simulink model "ieee30"  (R2017a)
settings: Solver=VariableStepDiscrete  StartTime=0.0  StopTime=0.012  MaxStep=1e-4  RelTol=1e-3
undefined symbols (not defined in the file): Angle, Magnitude
libraries: powerlib x548
(part 2 of 4)

== system ieee30/Bus1 ==
  G1 : powerlib/Measurements/Three-Phase V-I Measurement  VoltageMeasurement=no  SetLabelV=off  LabelV=V1  Vpu=off  VpuLL=off  CurrentMeasurement=no  SetLabelI=off  LabelI=I12  Ipu=off  Pbase=100e6  Vbase=500e3  OutputType=Complex  PhasorSimulation=on  PSBequivalent=0
  I13 : powerlib/Measurements/Three-Phase V-I Measurement  VoltageMeasurement=no  SetLabelV=off  LabelV=V1  Vpu=off  VpuLL=off  CurrentMeasurement=yes  SetLabelI=on  LabelI=I13  Ipu=off  Pbase=100e6  Vbase=500e3  OutputType=Magnitude-Angle  PhasorSimulation=on  PSBequivalent=0
  To Workspace2 : ToWorkspace  VariableName=I13  SaveFormat=Timeseries  SampleTime=0.01
  To Workspace3 : ToWorkspace  VariableName=I12  SaveFormat=Timeseries  SampleTime=0.01
  To Workspace4 : ToWorkspace  VariableName=V1  SaveFormat=Timeseries  SampleTime=0.01
  V1 I12 : powerlib/Measurements/Three-Phase V-I Measurement  VoltageMeasurement=phase-to-phase  SetLabelV=on  LabelV=V1  Vpu=off  VpuLL=off  CurrentMeasurement=yes  SetLabelI=on  LabelI=I12  Ipu=off  Pbase=100e6  Vbase=500e3  OutputType=Magnitude-Angle  PhasorSimulation=on  PSBequivalent=0
  G1A : PMIOPort  Port=1  Side=Left
  G1B : PMIOPort  Port=2  Side=Left
  G1C : PMIOPort  Port=3  Side=Left
  I13A : PMIOPort  Port=4  Side=Right
  I13B : PMIOPort  Port=5  Side=Right
  I13C : PMIOPort  Port=6  Side=Right
  I12C : PMIOPort  Port=7  Side=Right
  I12B : PMIOPort  Port=8  Side=Right
  I12A : PMIOPort  Port=9  Side=Right
  wires:
  [V1] -> To Workspace4/1
  [I12] -> To Workspace3/1
  [I13] -> To Workspace2/1
  connections:
  I13/LConn1 -- V1 I12/LConn1 -- G1/LConn1
  I13/LConn2 -- G1/LConn2 -- V1 I12/LConn2
  I13/LConn3 -- V1 I12/LConn3 -- G1/LConn3
  V1 I12/RConn1 -- I12A/RConn1
  V1 I12/RConn2 -- I12B/RConn1
  I12C/RConn1 -- V1 I12/RConn3
  I13/RConn3 -- I13C/RConn1
  I13/RConn1 -- I13A/RConn1
  I13/RConn2 -- I13B/RConn1
  G1B/RConn1 -- G1/RConn2
  G1A/RConn1 -- G1/RConn1
  G1C/RConn1 -- G1/RConn3

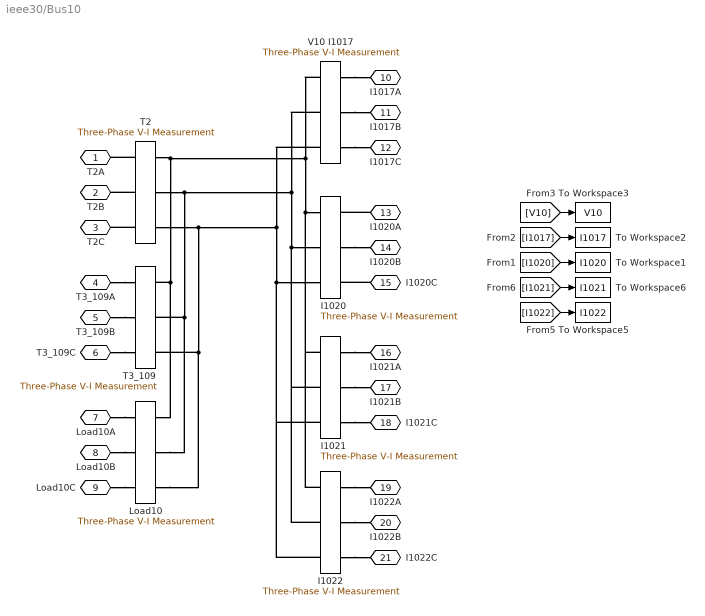
== system ieee30/Bus10 ==
  I1020 : powerlib/Measurements/Three-Phase V-I Measurement  VoltageMeasurement=no  SetLabelV=off  LabelV=V10  Vpu=off  VpuLL=off  CurrentMeasurement=yes  SetLabelI=on  LabelI=I1020  Ipu=off  Pbase=100e6  Vbase=500e3  OutputType=Magnitude-Angle  PhasorSimulation=on  PSBequivalent=0
  I1021 : powerlib/Measurements/Three-Phase V-I Measurement  VoltageMeasurement=no  SetLabelV=off  LabelV=V10  Vpu=off  VpuLL=off  CurrentMeasurement=yes  SetLabelI=on  LabelI=I1021  Ipu=off  Pbase=100e6  Vbase=500e3  OutputType=Magnitude-Angle  PhasorSimulation=on  PSBequivalent=0
  I1022 : powerlib/Measurements/Three-Phase V-I Measurement  VoltageMeasurement=no  SetLabelV=off  LabelV=V10  Vpu=off  VpuLL=off  CurrentMeasurement=yes  SetLabelI=on  LabelI=I1022  Ipu=off  Pbase=100e6  Vbase=500e3  OutputType=Magnitude-Angle  PhasorSimulation=on  PSBequivalent=0
  Load10 : powerlib/Measurements/Three-Phase V-I Measurement  VoltageMeasurement=no  SetLabelV=off  LabelV=Vabc  Vpu=off  VpuLL=off  CurrentMeasurement=no  SetLabelI=off  LabelI=Iabc  Ipu=off  Pbase=100e6  Vbase=500e3  OutputType=Complex  PhasorSimulation=on  PSBequivalent=0
  T2 : powerlib/Measurements/Three-Phase V-I Measurement  VoltageMeasurement=no  SetLabelV=off  LabelV=Vabc  Vpu=off  VpuLL=off  CurrentMeasurement=no  SetLabelI=off  LabelI=Iabc  Ipu=off  Pbase=100e6  Vbase=500e3  OutputType=Complex  PhasorSimulation=on  PSBequivalent=0
  T3_109 : powerlib/Measurements/Three-Phase V-I Measurement  VoltageMeasurement=no  SetLabelV=off  LabelV=Vabc  Vpu=off  VpuLL=off  CurrentMeasurement=no  SetLabelI=off  LabelI=Iabc  Ipu=off  Pbase=100e6  Vbase=500e3  OutputType=Complex  PhasorSimulation=on  PSBequivalent=0
  To Workspace1 : ToWorkspace  VariableName=I1020  SaveFormat=Timeseries  SampleTime=0.01
  To Workspace2 : ToWorkspace  VariableName=I1017  SaveFormat=Timeseries  SampleTime=0.01
  To Workspace3 : ToWorkspace  VariableName=V10  SaveFormat=Timeseries  SampleTime=0.01
  To Workspace5 : ToWorkspace  VariableName=I1022  SaveFormat=Timeseries  SampleTime=0.01
  To Workspace6 : ToWorkspace  VariableName=I1021  SaveFormat=Timeseries  SampleTime=0.01
  V10 I1017 : powerlib/Measurements/Three-Phase V-I Measurement  VoltageMeasurement=phase-to-phase  SetLabelV=on  LabelV=V10  Vpu=off  VpuLL=off  CurrentMeasurement=yes  SetLabelI=on  LabelI=I1017  Ipu=off  Pbase=100e6  Vbase=500e3  OutputType=Magnitude-Angle  PhasorSimulation=on  PSBequivalent=0
  T2A : PMIOPort  Port=1  Side=Left
  T2B : PMIOPort  Port=2  Side=Left
  T2C : PMIOPort  Port=3  Side=Left
  T3_109A : PMIOPort  Port=4  Side=Left
  T3_109B : PMIOPort  Port=5  Side=Left
  T3_109C : PMIOPort  Port=6  Side=Left
  Load10A : PMIOPort  Port=7  Side=Left
  Load10B : PMIOPort  Port=8  Side=Left
  Load10C : PMIOPort  Port=9  Side=Left
  I1017A : PMIOPort  Port=10  Side=Right
  I1017B : PMIOPort  Port=11  Side=Right
  I1017C : PMIOPort  Port=12  Side=Right
  I1020A : PMIOPort  Port=13  Side=Right
  I1020B : PMIOPort  Port=14  Side=Right
  I1020C : PMIOPort  Port=15  Side=Right
  I1021A : PMIOPort  Port=16  Side=Right
  I1021B : PMIOPort  Port=17  Side=Right
  I1021C : PMIOPort  Port=18  Side=Right
  I1022A : PMIOPort  Port=19  Side=Right
  I1022B : PMIOPort  Port=20  Side=Right
  I1022C : PMIOPort  Port=21  Side=Right
  wires:
  [I1020] -> To Workspace1/1
  [I1017] -> To Workspace2/1
  [I1022] -> To Workspace5/1
  [I1021] -> To Workspace6/1
  [V10] -> To Workspace3/1
  connections:
  T2/RConn3 -- T2C/RConn1
  T2/RConn1 -- T2A/RConn1
  T2/RConn2 -- T2B/RConn1
  T2/LConn1 -- I1022/LConn1 -- I1021/LConn1 -- I1020/LConn1 -- V10 I1017/LConn1 -- Load10/LConn1 -- T3_109/LConn1
  T2/LConn2 -- I1021/LConn2 -- I1022/LConn2 -- I1020/LConn2 -- V10 I1017/LConn2 -- Load10/LConn2 -- T3_109/LConn2
  T2/LConn3 -- Load10/LConn3 -- T3_109/LConn3 -- I1021/LConn3 -- I1022/LConn3 -- I1020/LConn3 -- V10 I1017/LConn3
  T3_109A/RConn1 -- T3_109/RConn1
  T3_109B/RConn1 -- T3_109/RConn2
  T3_109C/RConn1 -- T3_109/RConn3
  Load10C/RConn1 -- Load10/RConn3
  Load10B/RConn1 -- Load10/RConn2
  Load10A/RConn1 -- Load10/RConn1
  V10 I1017/RConn1 -- I1017A/RConn1
  V10 I1017/RConn3 -- I1017C/RConn1
  V10 I1017/RConn2 -- I1017B/RConn1
  I1020A/RConn1 -- I1020/RConn1
  I1020/RConn2 -- I1020B/RConn1
  I1020C/RConn1 -- I1020/RConn3
  I1021/RConn1 -- I1021A/RConn1
  I1021/RConn2 -- I1021B/RConn1
  I1021/RConn3 -- I1021C/RConn1
  I1022/RConn2 -- I1022B/RConn1
  I1022/RConn1 -- I1022A/RConn1
  I1022/RConn3 -- I1022C/RConn1

== system ieee30/Bus11 ==
  G11 : powerlib/Measurements/Three-Phase V-I Measurement  VoltageMeasurement=no  SetLabelV=off  LabelV=Vabc  Vpu=off  VpuLL=off  CurrentMeasurement=no  SetLabelI=off  LabelI=Iabc  Ipu=off  Pbase=100e6  Vbase=500e3  OutputType=Complex  PhasorSimulation=on  PSBequivalent=0
  T3_911 : powerlib/Measurements/Three-Phase V-I Measurement  VoltageMeasurement=no  SetLabelV=off  LabelV=Vabc  Vpu=off  VpuLL=off  CurrentMeasurement=no  SetLabelI=off  LabelI=Iabc  Ipu=off  Pbase=100e6  Vbase=500e3  OutputType=Complex  PhasorSimulation=on  PSBequivalent=0
  T3_911A : PMIOPort  Port=1  Side=Left
  T3_911B : PMIOPort  Port=2  Side=Left
  T3_911C : PMIOPort  Port=3  Side=Left
  G11A : PMIOPort  Port=4  Side=Right
  G11B : PMIOPort  Port=5  Side=Right
  G11C : PMIOPort  Port=6  Side=Right
  connections:
  T3_911/RConn1 -- T3_911A/RConn1
  T3_911/RConn2 -- T3_911B/RConn1
  G11/RConn3 -- G11C/RConn1
  G11/RConn2 -- G11B/RConn1
  G11/RConn1 -- G11A/RConn1
  T3_911/RConn3 -- T3_911C/RConn1
  T3_911/LConn1 -- G11/LConn1
  T3_911/LConn2 -- G11/LConn2
  T3_911/LConn3 -- G11/LConn3

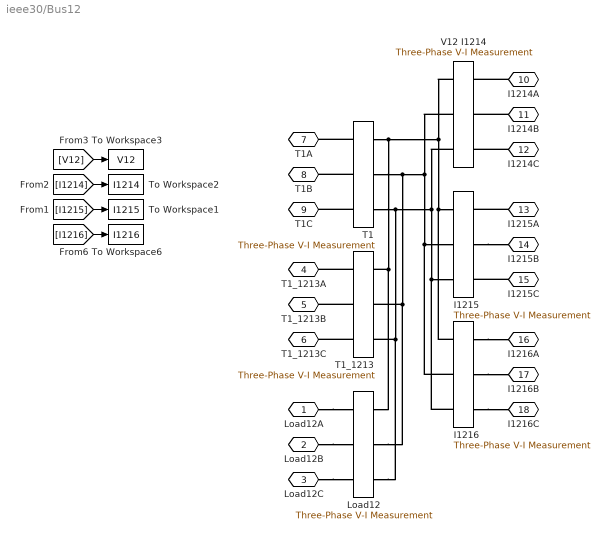
== system ieee30/Bus12 ==
  I1215 : powerlib/Measurements/Three-Phase V-I Measurement  VoltageMeasurement=no  SetLabelV=off  LabelV=V12  Vpu=off  VpuLL=off  CurrentMeasurement=yes  SetLabelI=on  LabelI=I1215  Ipu=off  Pbase=100e6  Vbase=500e3  OutputType=Magnitude-Angle  PhasorSimulation=on  PSBequivalent=0
  I1216 : powerlib/Measurements/Three-Phase V-I Measurement  VoltageMeasurement=no  SetLabelV=off  LabelV=V12  Vpu=off  VpuLL=off  CurrentMeasurement=yes  SetLabelI=on  LabelI=I1216  Ipu=off  Pbase=100e6  Vbase=500e3  OutputType=Magnitude-Angle  PhasorSimulation=on  PSBequivalent=0
  Load12 : powerlib/Measurements/Three-Phase V-I Measurement  VoltageMeasurement=no  SetLabelV=off  LabelV=V12  Vpu=off  VpuLL=off  CurrentMeasurement=no  SetLabelI=off  LabelI=I1214  Ipu=off  Pbase=100e6  Vbase=500e3  OutputType=Complex  PhasorSimulation=on  PSBequivalent=0
  T1 : powerlib/Measurements/Three-Phase V-I Measurement  VoltageMeasurement=no  SetLabelV=off  LabelV=V12  Vpu=off  VpuLL=off  CurrentMeasurement=no  SetLabelI=off  LabelI=I1214  Ipu=off  Pbase=100e6  Vbase=500e3  OutputType=Complex  PhasorSimulation=on  PSBequivalent=0
  T1_1213 : powerlib/Measurements/Three-Phase V-I Measurement  VoltageMeasurement=no  SetLabelV=off  LabelV=V12  Vpu=off  VpuLL=off  CurrentMeasurement=no  SetLabelI=off  LabelI=I1214  Ipu=off  Pbase=100e6  Vbase=500e3  OutputType=Complex  PhasorSimulation=on  PSBequivalent=0
  To Workspace1 : ToWorkspace  VariableName=I1215  SaveFormat=Timeseries  SampleTime=0.01
  To Workspace2 : ToWorkspace  VariableName=I1214  SaveFormat=Timeseries  SampleTime=0.01
  To Workspace3 : ToWorkspace  VariableName=V12  SaveFormat=Timeseries  SampleTime=0.01
  To Workspace6 : ToWorkspace  VariableName=I1216  SaveFormat=Timeseries  SampleTime=0.01
  V12 I1214 : powerlib/Measurements/Three-Phase V-I Measurement  VoltageMeasurement=phase-to-phase  SetLabelV=on  LabelV=V12  Vpu=off  VpuLL=off  CurrentMeasurement=yes  SetLabelI=on  LabelI=I1214  Ipu=off  Pbase=100e6  Vbase=500e3  OutputType=Magnitude-Angle  PhasorSimulation=on  PSBequivalent=0
  Load12A : PMIOPort  Port=1  Side=Left
  Load12B : PMIOPort  Port=2  Side=Left
  Load12C : PMIOPort  Port=3  Side=Left
  T1_1213A : PMIOPort  Port=4  Side=Left
  T1_1213B : PMIOPort  Port=5  Side=Left
  T1_1213C : PMIOPort  Port=6  Side=Left
  T1A : PMIOPort  Port=7  Side=Left
  T1B : PMIOPort  Port=8  Side=Left
  T1C : PMIOPort  Port=9  Side=Left
  I1214A : PMIOPort  Port=10  Side=Right
  I1214B : PMIOPort  Port=11  Side=Right
  I1214C : PMIOPort  Port=12  Side=Right
  I1215A : PMIOPort  Port=13  Side=Right
  I1215B : PMIOPort  Port=14  Side=Right
  I1215C : PMIOPort  Port=15  Side=Right
  I1216A : PMIOPort  Port=16  Side=Right
  I1216B : PMIOPort  Port=17  Side=Right
  I1216C : PMIOPort  Port=18  Side=Right
  wires:
  [I1215] -> To Workspace1/1
  [I1214] -> To Workspace2/1
  [I1216] -> To Workspace6/1
  [V12] -> To Workspace3/1
  connections:
  I1214C/RConn1 -- V12 I1214/RConn3
  I1214A/RConn1 -- V12 I1214/RConn1
  I1214B/RConn1 -- V12 I1214/RConn2
  T1/RConn2 -- T1B/RConn1
  T1/RConn3 -- T1C/RConn1
  T1/RConn1 -- T1A/RConn1
  T1/LConn1 -- Load12/LConn1 -- T1_1213/LConn1 -- I1216/LConn1 -- I1215/LConn1 -- V12 I1214/LConn1
  T1/LConn2 -- T1_1213/LConn2 -- Load12/LConn2 -- I1216/LConn2 -- I1215/LConn2 -- V12 I1214/LConn2
  T1/LConn3 -- I1216/LConn3 -- I1215/LConn3 -- V12 I1214/LConn3 -- T1_1213/LConn3 -- Load12/LConn3
  T1_1213/RConn3 -- T1_1213C/RConn1
  T1_1213/RConn2 -- T1_1213B/RConn1
  T1_1213/RConn1 -- T1_1213A/RConn1
  I1215A/RConn1 -- I1215/RConn1
  I1215/RConn2 -- I1215B/RConn1
  I1215C/RConn1 -- I1215/RConn3
  I1216/RConn1 -- I1216A/RConn1
  I1216/RConn3 -- I1216C/RConn1
  I1216/RConn2 -- I1216B/RConn1
  Load12A/RConn1 -- Load12/RConn1
  Load12B/RConn1 -- Load12/RConn2
  Load12C/RConn1 -- Load12/RConn3

== system ieee30/Bus13 ==
  G13 : powerlib/Measurements/Three-Phase V-I Measurement  VoltageMeasurement=no  SetLabelV=off  LabelV=Vabc  Vpu=off  VpuLL=off  CurrentMeasurement=no  SetLabelI=off  LabelI=Iabc  Ipu=off  Pbase=100e6  Vbase=500e3  OutputType=Complex  PhasorSimulation=on  PSBequivalent=0
  T1_1213 : powerlib/Measurements/Three-Phase V-I Measurement  VoltageMeasurement=no  SetLabelV=off  LabelV=Vabc  Vpu=off  VpuLL=off  CurrentMeasurement=no  SetLabelI=off  LabelI=Iabc  Ipu=off  Pbase=100e6  Vbase=500e3  OutputType=Complex  PhasorSimulation=on  PSBequivalent=0
  T1_1213A : PMIOPort  Port=1  Side=Left
  T1_1213B : PMIOPort  Port=2  Side=Left
  T1_1213C : PMIOPort  Port=3  Side=Left
  G13A : PMIOPort  Port=4  Side=Right
  G13B : PMIOPort  Port=5  Side=Right
  G13C : PMIOPort  Port=6  Side=Right
  connections:
  G13/RConn3 -- G13C/RConn1
  T1_1213/RConn3 -- T1_1213C/RConn1
  T1_1213/RConn1 -- T1_1213A/RConn1
  G13/RConn2 -- G13B/RConn1
  G13/RConn1 -- G13A/RConn1
  T1_1213/RConn2 -- T1_1213B/RConn1
  G13/LConn1 -- T1_1213/LConn1
  G13/LConn2 -- T1_1213/LConn2
  G13/LConn3 -- T1_1213/LConn3

== system ieee30/Bus14 ==
  I1415 : powerlib/Measurements/Three-Phase V-I Measurement  VoltageMeasurement=no  SetLabelV=off  LabelV=Vabc  Vpu=off  VpuLL=off  CurrentMeasurement=yes  SetLabelI=on  LabelI=I1415  Ipu=off  Pbase=100e6  Vbase=500e3  OutputType=Magnitude-Angle  PhasorSimulation=on  PSBequivalent=0
  Load14 : powerlib/Measurements/Three-Phase V-I Measurement  VoltageMeasurement=no  SetLabelV=off  LabelV=Vabc  Vpu=off  VpuLL=off  CurrentMeasurement=no  SetLabelI=off  LabelI=I1415  Ipu=off  Pbase=100e6  Vbase=500e3  OutputType=Complex  PhasorSimulation=on  PSBequivalent=0
  To Workspace1 : ToWorkspace  VariableName=I1415  SaveFormat=Timeseries  SampleTime=0.01
  To Workspace2 : ToWorkspace  VariableName=I1412  SaveFormat=Timeseries  SampleTime=0.01
  To Workspace3 : ToWorkspace  VariableName=V14  SaveFormat=Timeseries  SampleTime=0.01
  V14 I1412 : powerlib/Measurements/Three-Phase V-I Measurement  VoltageMeasurement=phase-to-phase  SetLabelV=on  LabelV=V14  Vpu=off  VpuLL=off  CurrentMeasurement=yes  SetLabelI=on  LabelI=I1412  Ipu=off  Pbase=100e6  Vbase=500e3  OutputType=Magnitude-Angle  PhasorSimulation=on  PSBequivalent=0
  Load14A : PMIOPort  Port=1  Side=Left
  Load14B : PMIOPort  Port=2  Side=Left
  Load14C : PMIOPort  Port=3  Side=Left
  I1412A : PMIOPort  Port=4  Side=Left
  I1412B : PMIOPort  Port=5  Side=Left
  I1412C : PMIOPort  Port=6  Side=Left
  I1415A : PMIOPort  Port=7  Side=Right
  I1415B : PMIOPort  Port=8  Side=Right
  I1415C : PMIOPort  Port=9  Side=Right
  wires:
  [V14] -> To Workspace3/1
  [I1415] -> To Workspace1/1
  [I1412] -> To Workspace2/1
  connections:
  I1415/RConn3 -- I1415C/RConn1
  V14 I1412/RConn3 -- I1412C/RConn1
  V14 I1412/RConn2 -- I1412B/RConn1
  I1415/RConn2 -- I1415B/RConn1
  V14 I1412/RConn1 -- I1412A/RConn1
  I1415/RConn1 -- I1415A/RConn1
  V14 I1412/LConn1 -- Load14/LConn1 -- I1415/LConn1
  V14 I1412/LConn2 -- I1415/LConn2 -- Load14/LConn2
  V14 I1412/LConn3 -- I1415/LConn3 -- Load14/LConn3
  Load14A/RConn1 -- Load14/RConn1
  Load14/RConn2 -- Load14B/RConn1
  Load14C/RConn1 -- Load14/RConn3

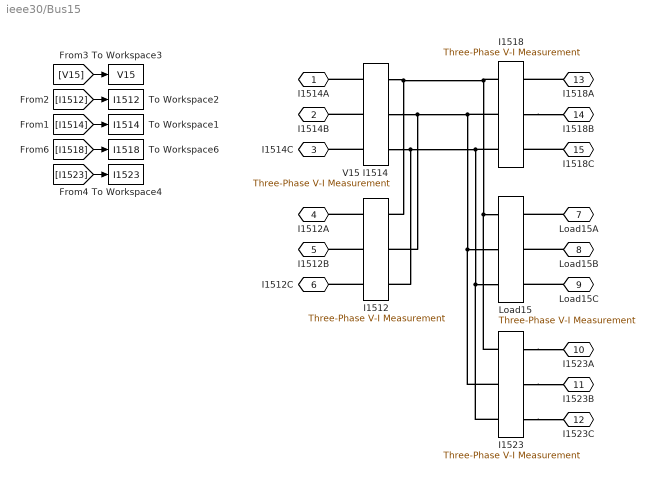
== system ieee30/Bus15 ==
  I1512 : powerlib/Measurements/Three-Phase V-I Measurement  VoltageMeasurement=no  SetLabelV=off  LabelV=V15  Vpu=off  VpuLL=off  CurrentMeasurement=yes  SetLabelI=on  LabelI=I1512  Ipu=off  Pbase=100e6  Vbase=500e3  OutputType=Magnitude-Angle  PhasorSimulation=on  PSBequivalent=0
  I1518 : powerlib/Measurements/Three-Phase V-I Measurement  VoltageMeasurement=no  SetLabelV=off  LabelV=Vabc  Vpu=off  VpuLL=off  CurrentMeasurement=yes  SetLabelI=on  LabelI=I1518  Ipu=off  Pbase=100e6  Vbase=500e3  OutputType=Magnitude-Angle  PhasorSimulation=on  PSBequivalent=0
  I1523 : powerlib/Measurements/Three-Phase V-I Measurement  VoltageMeasurement=no  SetLabelV=off  LabelV=Vabc  Vpu=off  VpuLL=off  CurrentMeasurement=yes  SetLabelI=on  LabelI=I1523  Ipu=off  Pbase=100e6  Vbase=500e3  OutputType=Magnitude-Angle  PhasorSimulation=on  PSBequivalent=0
  Load15 : powerlib/Measurements/Three-Phase V-I Measurement  VoltageMeasurement=no  SetLabelV=off  LabelV=Vabc  Vpu=off  VpuLL=off  CurrentMeasurement=no  SetLabelI=off  LabelI=Iabc  Ipu=off  Pbase=100e6  Vbase=500e3  OutputType=Complex  PhasorSimulation=on  PSBequivalent=0
  To Workspace1 : ToWorkspace  VariableName=I1514  SaveFormat=Timeseries  SampleTime=0.01
  To Workspace2 : ToWorkspace  VariableName=I1512  SaveFormat=Timeseries  SampleTime=0.01
  To Workspace3 : ToWorkspace  VariableName=V15  SaveFormat=Timeseries  SampleTime=0.01
  To Workspace4 : ToWorkspace  VariableName=I1523  SaveFormat=Timeseries  SampleTime=0.01
  To Workspace6 : ToWorkspace  VariableName=I1518  SaveFormat=Timeseries  SampleTime=0.01
  V15 I1514 : powerlib/Measurements/Three-Phase V-I Measurement  VoltageMeasurement=phase-to-phase  SetLabelV=on  LabelV=V15  Vpu=off  VpuLL=off  CurrentMeasurement=yes  SetLabelI=on  LabelI=I1514  Ipu=off  Pbase=100e6  Vbase=500e3  OutputType=Magnitude-Angle  PhasorSimulation=on  PSBequivalent=0
  I1514A : PMIOPort  Port=1  Side=Left
  I1514B : PMIOPort  Port=2  Side=Left
  I1514C : PMIOPort  Port=3  Side=Left
  I1512A : PMIOPort  Port=4  Side=Left
  I1512B : PMIOPort  Port=5  Side=Left
  I1512C : PMIOPort  Port=6  Side=Left
  Load15A : PMIOPort  Port=7  Side=Right
  Load15B : PMIOPort  Port=8  Side=Right
  Load15C : PMIOPort  Port=9  Side=Right
  I1523A : PMIOPort  Port=10  Side=Right
  I1523B : PMIOPort  Port=11  Side=Right
  I1523C : PMIOPort  Port=12  Side=Right
  I1518A : PMIOPort  Port=13  Side=Left
  I1518B : PMIOPort  Port=14  Side=Left
  I1518C : PMIOPort  Port=15  Side=Left
  wires:
  [I1518] -> To Workspace6/1
  [V15] -> To Workspace3/1
  [I1514] -> To Workspace1/1
  [I1512] -> To Workspace2/1
  [I1523] -> To Workspace4/1
  connections:
  V15 I1514/RConn1 -- I1514A/RConn1
  V15 I1514/RConn3 -- I1514C/RConn1
  V15 I1514/RConn2 -- I1514B/RConn1
  V15 I1514/LConn1 -- I1523/LConn1 -- Load15/LConn1 -- I1518/LConn1 -- I1512/LConn1
  V15 I1514/LConn2 -- I1512/LConn2 -- I1523/LConn2 -- Load15/LConn2 -- I1518/LConn2
  V15 I1514/LConn3 -- I1512/LConn3 -- I1523/LConn3 -- Load15/LConn3 -- I1518/LConn3
  I1512/RConn3 -- I1512C/RConn1
  I1512/RConn1 -- I1512A/RConn1
  I1512/RConn2 -- I1512B/RConn1
  Load15A/RConn1 -- Load15/RConn1
  Load15B/RConn1 -- Load15/RConn2
  Load15C/RConn1 -- Load15/RConn3
  I1523/RConn1 -- I1523A/RConn1
  I1523/RConn3 -- I1523C/RConn1
  I1523/RConn2 -- I1523B/RConn1
  I1518A/RConn1 -- I1518/RConn1
  I1518/RConn2 -- I1518B/RConn1
  I1518C/RConn1 -- I1518/RConn3

== system ieee30/Bus16 ==
  I1617 : powerlib/Measurements/Three-Phase V-I Measurement  VoltageMeasurement=no  SetLabelV=off  LabelV=Vabc  Vpu=off  VpuLL=off  CurrentMeasurement=yes  SetLabelI=on  LabelI=I1617  Ipu=off  Pbase=100e6  Vbase=500e3  OutputType=Magnitude-Angle  PhasorSimulation=on  PSBequivalent=0
  Load16 : powerlib/Measurements/Three-Phase V-I Measurement  VoltageMeasurement=no  SetLabelV=off  LabelV=Vabc  Vpu=off  VpuLL=off  CurrentMeasurement=no  SetLabelI=off  LabelI=Iabc  Ipu=off  Pbase=100e6  Vbase=500e3  OutputType=Complex  PhasorSimulation=on  PSBequivalent=0
  To Workspace1 : ToWorkspace  VariableName=I1617  SaveFormat=Timeseries  SampleTime=0.01
  To Workspace2 : ToWorkspace  VariableName=I1612  SaveFormat=Timeseries  SampleTime=0.01
  To Workspace6 : ToWorkspace  VariableName=V16  SaveFormat=Timeseries  SampleTime=0.01
  V16 I1612 : powerlib/Measurements/Three-Phase V-I Measurement  VoltageMeasurement=phase-to-phase  SetLabelV=on  LabelV=V16  Vpu=off  VpuLL=off  CurrentMeasurement=yes  SetLabelI=on  LabelI=I1612  Ipu=off  Pbase=100e6  Vbase=500e3  OutputType=Magnitude-Angle  PhasorSimulation=on  PSBequivalent=0
  I1612A : PMIOPort  Port=1  Side=Left
  I1612B : PMIOPort  Port=2  Side=Left
  I1612C : PMIOPort  Port=3  Side=Left
  I1617A : PMIOPort  Port=4  Side=Left
  I1617B : PMIOPort  Port=5  Side=Left
  I1617C : PMIOPort  Port=6  Side=Left
  Load16A : PMIOPort  Port=7  Side=Right
  Load16B : PMIOPort  Port=8  Side=Right
  Load16C : PMIOPort  Port=9  Side=Right
  wires:
  [V16] -> To Workspace6/1
  [I1617] -> To Workspace1/1
  [I1612] -> To Workspace2/1
  connections:
  V16 I1612/RConn1 -- I1612A/RConn1
  V16 I1612/RConn2 -- I1612B/RConn1
  V16 I1612/RConn3 -- I1612C/RConn1
  V16 I1612/LConn1 -- I1617/LConn1 -- Load16/LConn1
  V16 I1612/LConn2 -- I1617/LConn2 -- Load16/LConn2
  V16 I1612/LConn3 -- I1617/LConn3 -- Load16/LConn3
  I1617/RConn1 -- I1617A/RConn1
  I1617/RConn2 -- I1617B/RConn1
  I1617/RConn3 -- I1617C/RConn1
  Load16A/RConn1 -- Load16/RConn1
  Load16B/RConn1 -- Load16/RConn2
  Load16C/RConn1 -- Load16/RConn3

== system ieee30/Bus17 ==
  I1710 : powerlib/Measurements/Three-Phase V-I Measurement  VoltageMeasurement=no  SetLabelV=off  LabelV=Vabc  Vpu=off  VpuLL=off  CurrentMeasurement=yes  SetLabelI=on  LabelI=I1710  Ipu=off  Pbase=100e6  Vbase=500e3  OutputType=Magnitude-Angle  PhasorSimulation=on  PSBequivalent=0
  Load17 : powerlib/Measurements/Three-Phase V-I Measurement  VoltageMeasurement=no  SetLabelV=off  LabelV=Vabc  Vpu=off  VpuLL=off  CurrentMeasurement=no  SetLabelI=off  LabelI=Iabc  Ipu=off  Pbase=100e6  Vbase=500e3  OutputType=Complex  PhasorSimulation=on  PSBequivalent=0
  To Workspace1 : ToWorkspace  VariableName=I1716  SaveFormat=Timeseries  SampleTime=0.01
  To Workspace2 : ToWorkspace  VariableName=I1710  SaveFormat=Timeseries  SampleTime=0.01
  To Workspace6 : ToWorkspace  VariableName=V17  SaveFormat=Timeseries  SampleTime=0.01
  V17 I1716 : powerlib/Measurements/Three-Phase V-I Measurement  VoltageMeasurement=phase-to-phase  SetLabelV=on  LabelV=V17  Vpu=off  VpuLL=off  CurrentMeasurement=yes  SetLabelI=on  LabelI=I1716  Ipu=off  Pbase=100e6  Vbase=500e3  OutputType=Magnitude-Angle  PhasorSimulation=on  PSBequivalent=0
  I1716A : PMIOPort  Port=1  Side=Left
  I1716B : PMIOPort  Port=2  Side=Left
  I1716C : PMIOPort  Port=3  Side=Left
  I1710A : PMIOPort  Port=4  Side=Left
  I1710B : PMIOPort  Port=5  Side=Left
  I1710C : PMIOPort  Port=6  Side=Left
  Load17A : PMIOPort  Port=7  Side=Right
  Load17B : PMIOPort  Port=8  Side=Right
  Load17C : PMIOPort  Port=9  Side=Right
  wires:
  [V17] -> To Workspace6/1
  [I1716] -> To Workspace1/1
  [I1710] -> To Workspace2/1
  connections:
  V17 I1716/RConn1 -- I1716A/RConn1
  V17 I1716/RConn2 -- I1716B/RConn1
  V17 I1716/RConn3 -- I1716C/RConn1
  V17 I1716/LConn1 -- Load17/LConn1 -- I1710/LConn1
  V17 I1716/LConn2 -- Load17/LConn2 -- I1710/LConn2
  V17 I1716/LConn3 -- Load17/LConn3 -- I1710/LConn3
  I1710/RConn1 -- I1710A/RConn1
  I1710/RConn2 -- I1710B/RConn1
  I1710/RConn3 -- I1710C/RConn1
  Load17A/RConn1 -- Load17/RConn1
  Load17B/RConn1 -- Load17/RConn2
  Load17C/RConn1 -- Load17/RConn3

== system ieee30/Bus18 ==
  I1819 : powerlib/Measurements/Three-Phase V-I Measurement  VoltageMeasurement=no  SetLabelV=off  LabelV=Vabc  Vpu=off  VpuLL=off  CurrentMeasurement=yes  SetLabelI=on  LabelI=I1819  Ipu=off  Pbase=100e6  Vbase=500e3  OutputType=Magnitude-Angle  PhasorSimulation=on  PSBequivalent=0
  Load18 : powerlib/Measurements/Three-Phase V-I Measurement  VoltageMeasurement=no  SetLabelV=off  LabelV=Vabc  Vpu=off  VpuLL=off  CurrentMeasurement=no  SetLabelI=off  LabelI=Iabc  Ipu=off  Pbase=100e6  Vbase=500e3  OutputType=Complex  PhasorSimulation=on  PSBequivalent=0
  To Workspace1 : ToWorkspace  VariableName=I1819  SaveFormat=Timeseries  SampleTime=0.01
  To Workspace2 : ToWorkspace  VariableName=I1815  SaveFormat=Timeseries  SampleTime=0.01
  To Workspace6 : ToWorkspace  VariableName=V18  SaveFormat=Timeseries  SampleTime=0.01
  V18 I1815 : powerlib/Measurements/Three-Phase V-I Measurement  VoltageMeasurement=phase-to-phase  SetLabelV=on  LabelV=V18  Vpu=off  VpuLL=off  CurrentMeasurement=yes  SetLabelI=on  LabelI=I1815  Ipu=off  Pbase=100e6  Vbase=500e3  OutputType=Magnitude-Angle  PhasorSimulation=on  PSBequivalent=0
  I1815A : PMIOPort  Port=1  Side=Left
  I1815B : PMIOPort  Port=2  Side=Left
  I1815C : PMIOPort  Port=3  Side=Left
  I1819A : PMIOPort  Port=4  Side=Left
  I1819B : PMIOPort  Port=5  Side=Left
  I1819C : PMIOPort  Port=6  Side=Left
  Load18A : PMIOPort  Port=7  Side=Right
  Load18B : PMIOPort  Port=8  Side=Right
  Load18C : PMIOPort  Port=9  Side=Right
  wires:
  [V18] -> To Workspace6/1
  [I1815] -> To Workspace2/1
  [I1819] -> To Workspace1/1
  connections:
  I1819/RConn2 -- I1819B/RConn1
  I1819/RConn3 -- I1819C/RConn1
  I1819/RConn1 -- I1819A/RConn1
  V18 I1815/RConn2 -- I1815B/RConn1
  V18 I1815/RConn1 -- I1815A/RConn1
  V18 I1815/RConn3 -- I1815C/RConn1
  V18 I1815/LConn1 -- Load18/LConn1 -- I1819/LConn1
  V18 I1815/LConn2 -- Load18/LConn2 -- I1819/LConn2
  V18 I1815/LConn3 -- Load18/LConn3 -- I1819/LConn3
  Load18/RConn1 -- Load18A/RConn1
  Load18/RConn3 -- Load18C/RConn1
  Load18/RConn2 -- Load18B/RConn1

== system ieee30/Bus19 ==
  I1920 : powerlib/Measurements/Three-Phase V-I Measurement  VoltageMeasurement=no  SetLabelV=off  LabelV=Vabc  Vpu=off  VpuLL=off  CurrentMeasurement=yes  SetLabelI=on  LabelI=I1920  Ipu=off  Pbase=100e6  Vbase=500e3  OutputType=Magnitude-Angle  PhasorSimulation=on  PSBequivalent=0
  Load19 : powerlib/Measurements/Three-Phase V-I Measurement  VoltageMeasurement=no  SetLabelV=off  LabelV=Vabc  Vpu=off  VpuLL=off  CurrentMeasurement=no  SetLabelI=off  LabelI=Iabc  Ipu=off  Pbase=100e6  Vbase=500e3  OutputType=Complex  PhasorSimulation=on  PSBequivalent=0
  To Workspace1 : ToWorkspace  VariableName=I1920  SaveFormat=Timeseries  SampleTime=0.01
  To Workspace2 : ToWorkspace  VariableName=I1918  SaveFormat=Timeseries  SampleTime=0.01
  To Workspace6 : ToWorkspace  VariableName=V19  SaveFormat=Timeseries  SampleTime=0.01
  V19 I1918 : powerlib/Measurements/Three-Phase V-I Measurement  VoltageMeasurement=phase-to-phase  SetLabelV=on  LabelV=V19  Vpu=off  VpuLL=off  CurrentMeasurement=yes  SetLabelI=on  LabelI=I1918  Ipu=off  Pbase=100e6  Vbase=500e3  OutputType=Magnitude-Angle  PhasorSimulation=on  PSBequivalent=0
  I1918A : PMIOPort  Port=1  Side=Left
  I1918B : PMIOPort  Port=2  Side=Left
  I1918C : PMIOPort  Port=3  Side=Left
  I1920A : PMIOPort  Port=4  Side=Left
  I1920B : PMIOPort  Port=5  Side=Left
  I1920C : PMIOPort  Port=6  Side=Left
  Load19A : PMIOPort  Port=7  Side=Right
  Load19B : PMIOPort  Port=8  Side=Right
  Load19C : PMIOPort  Port=9  Side=Right
  wires:
  [V19] -> To Workspace6/1
  [I1918] -> To Workspace2/1
  [I1920] -> To Workspace1/1
  connections:
  V19 I1918/RConn1 -- I1918A/RConn1
  V19 I1918/RConn3 -- I1918C/RConn1
  V19 I1918/RConn2 -- I1918B/RConn1
  V19 I1918/LConn1 -- Load19/LConn1 -- I1920/LConn1
  V19 I1918/LConn2 -- Load19/LConn2 -- I1920/LConn2
  V19 I1918/LConn3 -- Load19/LConn3 -- I1920/LConn3
  I1920/RConn1 -- I1920A/RConn1
  I1920B/RConn1 -- I1920/RConn2
  I1920/RConn3 -- I1920C/RConn1
  Load19A/RConn1 -- Load19/RConn1
  Load19B/RConn1 -- Load19/RConn2
  Load19C/RConn1 -- Load19/RConn3

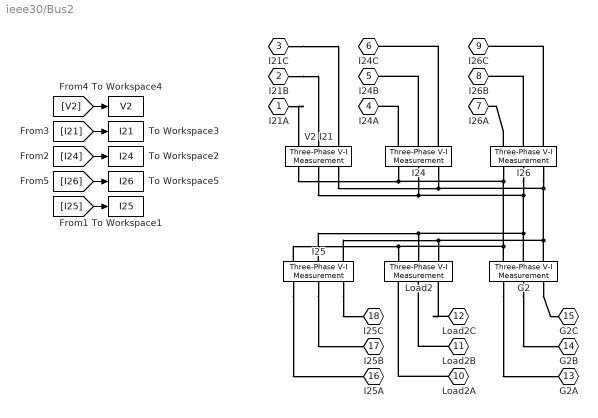
== system ieee30/Bus2 ==
  G2 : powerlib/Measurements/Three-Phase V-I Measurement  VoltageMeasurement=no  SetLabelV=off  LabelV=V2  Vpu=off  VpuLL=off  CurrentMeasurement=no  SetLabelI=on  LabelI=I25  Ipu=off  Pbase=100e6  Vbase=500e3  OutputType=Complex  PhasorSimulation=on  PSBequivalent=0
  I24 : powerlib/Measurements/Three-Phase V-I Measurement  VoltageMeasurement=no  SetLabelV=off  LabelV=V2  Vpu=off  VpuLL=off  CurrentMeasurement=yes  SetLabelI=on  LabelI=I24  Ipu=off  Pbase=100e6  Vbase=500e3  OutputType=Magnitude-Angle  PhasorSimulation=on  PSBequivalent=0
  I25 : powerlib/Measurements/Three-Phase V-I Measurement  VoltageMeasurement=no  SetLabelV=off  LabelV=V2  Vpu=off  VpuLL=off  CurrentMeasurement=yes  SetLabelI=on  LabelI=I25  Ipu=off  Pbase=100e6  Vbase=500e3  OutputType=Magnitude-Angle  PhasorSimulation=on  PSBequivalent=0
  I26 : powerlib/Measurements/Three-Phase V-I Measurement  VoltageMeasurement=no  SetLabelV=off  LabelV=V2  Vpu=off  VpuLL=off  CurrentMeasurement=yes  SetLabelI=on  LabelI=I26  Ipu=off  Pbase=100e6  Vbase=500e3  OutputType=Magnitude-Angle  PhasorSimulation=on  PSBequivalent=0
  Load2 : powerlib/Measurements/Three-Phase V-I Measurement  VoltageMeasurement=no  SetLabelV=off  LabelV=V2  Vpu=off  VpuLL=off  CurrentMeasurement=no  SetLabelI=off  LabelI=I25  Ipu=off  Pbase=100e6  Vbase=500e3  OutputType=Complex  PhasorSimulation=on  PSBequivalent=0
  To Workspace1 : ToWorkspace  VariableName=I25  SaveFormat=Timeseries  SampleTime=0.01
  To Workspace2 : ToWorkspace  VariableName=I24  SaveFormat=Timeseries  SampleTime=0.01
  To Workspace3 : ToWorkspace  VariableName=I21  SaveFormat=Timeseries  SampleTime=0.01
  To Workspace4 : ToWorkspace  VariableName=V2  SaveFormat=Timeseries  SampleTime=0.01
  To Workspace5 : ToWorkspace  VariableName=I26  SaveFormat=Timeseries  SampleTime=0.01
  V2 I21 : powerlib/Measurements/Three-Phase V-I Measurement  VoltageMeasurement=phase-to-phase  SetLabelV=on  LabelV=V2  Vpu=off  VpuLL=off  CurrentMeasurement=yes  SetLabelI=on  LabelI=I21  Ipu=off  Pbase=100e6  Vbase=500e3  OutputType=Magnitude-Angle  PhasorSimulation=on  PSBequivalent=0
  I21A : PMIOPort  Port=1  Side=Left
  I21B : PMIOPort  Port=2  Side=Left
  I21C : PMIOPort  Port=3  Side=Left
  I24A : PMIOPort  Port=4  Side=Left
  I24B : PMIOPort  Port=5  Side=Left
  I24C : PMIOPort  Port=6  Side=Left
  I26A : PMIOPort  Port=7  Side=Left
  I26B : PMIOPort  Port=8  Side=Left
  I26C : PMIOPort  Port=9  Side=Left
  Load2A : PMIOPort  Port=10  Side=Right
  Load2B : PMIOPort  Port=11  Side=Right
  Load2C : PMIOPort  Port=12  Side=Right
  G2A : PMIOPort  Port=13  Side=Right
  G2B : PMIOPort  Port=14  Side=Right
  G2C : PMIOPort  Port=15  Side=Right
  I25A : PMIOPort  Port=16  Side=Right
  I25B : PMIOPort  Port=17  Side=Right
  I25C : PMIOPort  Port=18  Side=Right
  wires:
  [V2] -> To Workspace4/1
  [I21] -> To Workspace3/1
  [I24] -> To Workspace2/1
  [I25] -> To Workspace1/1
  [I26] -> To Workspace5/1
  connections:
  Load2/LConn1 -- I25/LConn1 -- V2 I21/LConn1 -- I24/LConn1 -- I26/LConn1 -- G2/LConn1
  Load2/LConn2 -- I26/LConn2 -- V2 I21/LConn2 -- I24/LConn2 -- G2/LConn2 -- I25/LConn2
  Load2/LConn3 -- I25/LConn3 -- G2/LConn3 -- I26/LConn3 -- V2 I21/LConn3 -- I24/LConn3
  I21A/RConn1 -- V2 I21/RConn1
  I21B/RConn1 -- V2 I21/RConn2
  I21C/RConn1 -- V2 I21/RConn3
  I24/RConn2 -- I24B/RConn1
  I24/RConn1 -- I24A/RConn1
  I24/RConn3 -- I24C/RConn1
  I26/RConn3 -- I26C/RConn1
  I26/RConn1 -- I26A/RConn1
  I26/RConn2 -- I26B/RConn1
  I25/RConn3 -- I25C/RConn1
  I25/RConn2 -- I25B/RConn1
  I25/RConn1 -- I25A/RConn1
  Load2A/RConn1 -- Load2/RConn1
  Load2B/RConn1 -- Load2/RConn2
  Load2C/RConn1 -- Load2/RConn3
  G2/RConn1 -- G2A/RConn1
  G2/RConn3 -- G2C/RConn1
  G2/RConn2 -- G2B/RConn1

== system ieee30/Bus20 ==
  I2010 : powerlib/Measurements/Three-Phase V-I Measurement  VoltageMeasurement=no  SetLabelV=off  LabelV=Vabc  Vpu=off  VpuLL=off  CurrentMeasurement=yes  SetLabelI=on  LabelI=I2010  Ipu=off  Pbase=100e6  Vbase=500e3  OutputType=Magnitude-Angle  PhasorSimulation=on  PSBequivalent=0
  Load20 : powerlib/Measurements/Three-Phase V-I Measurement  VoltageMeasurement=no  SetLabelV=off  LabelV=Vabc  Vpu=off  VpuLL=off  CurrentMeasurement=no  SetLabelI=off  LabelI=Iabc  Ipu=off  Pbase=100e6  Vbase=500e3  OutputType=Complex  PhasorSimulation=on  PSBequivalent=0
  To Workspace1 : ToWorkspace  VariableName=I2019  SaveFormat=Timeseries  SampleTime=0.01
  To Workspace2 : ToWorkspace  VariableName=I2010  SaveFormat=Timeseries  SampleTime=0.01
  To Workspace6 : ToWorkspace  VariableName=V20  SaveFormat=Timeseries  SampleTime=0.01
  V20 I2019 : powerlib/Measurements/Three-Phase V-I Measurement  VoltageMeasurement=phase-to-phase  SetLabelV=on  LabelV=V20  Vpu=off  VpuLL=off  CurrentMeasurement=yes  SetLabelI=on  LabelI=I2019  Ipu=off  Pbase=100e6  Vbase=500e3  OutputType=Magnitude-Angle  PhasorSimulation=on  PSBequivalent=0
  I2019A : PMIOPort  Port=1  Side=Left
  I2019B : PMIOPort  Port=2  Side=Left
  I2019C : PMIOPort  Port=3  Side=Left
  I2010A : PMIOPort  Port=4  Side=Left
  I2010B : PMIOPort  Port=5  Side=Left
  I2010C : PMIOPort  Port=6  Side=Left
  Load20A : PMIOPort  Port=7  Side=Right
  Load20B : PMIOPort  Port=8  Side=Right
  Load20C : PMIOPort  Port=9  Side=Right
  wires:
  [V20] -> To Workspace6/1
  [I2010] -> To Workspace2/1
  [I2019] -> To Workspace1/1
  connections:
  V20 I2019/RConn1 -- I2019A/RConn1
  V20 I2019/RConn2 -- I2019B/RConn1
  V20 I2019/RConn3 -- I2019C/RConn1
  V20 I2019/LConn1 -- Load20/LConn1 -- I2010/LConn1
  V20 I2019/LConn2 -- Load20/LConn2 -- I2010/LConn2
  V20 I2019/LConn3 -- Load20/LConn3 -- I2010/LConn3
  I2010/RConn1 -- I2010A/RConn1
  I2010/RConn2 -- I2010B/RConn1
  I2010/RConn3 -- I2010C/RConn1
  Load20A/RConn1 -- Load20/RConn1
  Load20B/RConn1 -- Load20/RConn2
  Load20C/RConn1 -- Load20/RConn3

== system ieee30/Bus21 ==
  I2122 : powerlib/Measurements/Three-Phase V-I Measurement  VoltageMeasurement=no  SetLabelV=off  LabelV=V21  Vpu=off  VpuLL=off  CurrentMeasurement=yes  SetLabelI=on  LabelI=I2122  Ipu=off  Pbase=100e6  Vbase=500e3  OutputType=Magnitude-Angle  PhasorSimulation=on  PSBequivalent=0
  Load21 : powerlib/Measurements/Three-Phase V-I Measurement  VoltageMeasurement=no  SetLabelV=off  LabelV=Vabc  Vpu=off  VpuLL=off  CurrentMeasurement=no  SetLabelI=off  LabelI=Iabc  Ipu=off  Pbase=100e6  Vbase=500e3  OutputType=Complex  PhasorSimulation=on  PSBequivalent=0
  To Workspace1 : ToWorkspace  VariableName=I2122  SaveFormat=Timeseries  SampleTime=0.01
  To Workspace2 : ToWorkspace  VariableName=I2110  SaveFormat=Timeseries  SampleTime=0.01
  To Workspace6 : ToWorkspace  VariableName=V21  SaveFormat=Timeseries  SampleTime=0.01
  V21 I2110 : powerlib/Measurements/Three-Phase V-I Measurement  VoltageMeasurement=phase-to-phase  SetLabelV=on  LabelV=V21  Vpu=off  VpuLL=off  CurrentMeasurement=yes  SetLabelI=on  LabelI=I2110  Ipu=off  Pbase=100e6  Vbase=500e3  OutputType=Magnitude-Angle  PhasorSimulation=on  PSBequivalent=0
  I2110A : PMIOPort  Port=1  Side=Left
  I2110B : PMIOPort  Port=2  Side=Left
  I2110C : PMIOPort  Port=3  Side=Left
  I2122A : PMIOPort  Port=4  Side=Left
  I2122B : PMIOPort  Port=5  Side=Left
  I2122C : PMIOPort  Port=6  Side=Left
  Load21A : PMIOPort  Port=7  Side=Right
  Load21B : PMIOPort  Port=8  Side=Right
  Load21C : PMIOPort  Port=9  Side=Right
  wires:
  [V21] -> To Workspace6/1
  [I2110] -> To Workspace2/1
  [I2122] -> To Workspace1/1
  connections:
  V21 I2110/RConn2 -- I2110B/RConn1
  Load21/RConn1 -- Load21A/RConn1
  V21 I2110/RConn1 -- I2110A/RConn1
  Load21/RConn2 -- Load21B/RConn1
  Load21/RConn3 -- Load21C/RConn1
  V21 I2110/RConn3 -- I2110C/RConn1
  V21 I2110/LConn1 -- I2122/LConn1 -- Load21/LConn1
  V21 I2110/LConn2 -- I2122/LConn2 -- Load21/LConn2
  V21 I2110/LConn3 -- I2122/LConn3 -- Load21/LConn3
  I2122/RConn1 -- I2122A/RConn1
  I2122/RConn2 -- I2122B/RConn1
  I2122/RConn3 -- I2122C/RConn1

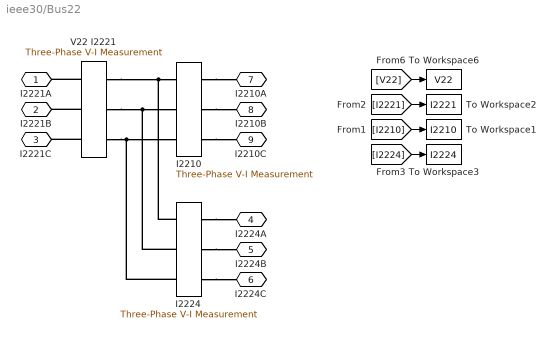
== system ieee30/Bus22 ==
  I2210 : powerlib/Measurements/Three-Phase V-I Measurement  VoltageMeasurement=no  SetLabelV=off  LabelV=Vabc  Vpu=off  VpuLL=off  CurrentMeasurement=yes  SetLabelI=on  LabelI=I2210  Ipu=off  Pbase=100e6  Vbase=500e3  OutputType=Magnitude-Angle  PhasorSimulation=on  PSBequivalent=0
  I2224 : powerlib/Measurements/Three-Phase V-I Measurement  VoltageMeasurement=no  SetLabelV=off  LabelV=V21  Vpu=off  VpuLL=off  CurrentMeasurement=yes  SetLabelI=on  LabelI=I2224  Ipu=off  Pbase=100e6  Vbase=500e3  OutputType=Magnitude-Angle  PhasorSimulation=on  PSBequivalent=0
  To Workspace1 : ToWorkspace  VariableName=I2210  SaveFormat=Timeseries  SampleTime=0.01
  To Workspace2 : ToWorkspace  VariableName=I2221  SaveFormat=Timeseries  SampleTime=0.01
  To Workspace3 : ToWorkspace  VariableName=I2224  SaveFormat=Timeseries  SampleTime=0.01
  To Workspace6 : ToWorkspace  VariableName=V22  SaveFormat=Timeseries  SampleTime=0.01
  V22 I2221 : powerlib/Measurements/Three-Phase V-I Measurement  VoltageMeasurement=phase-to-phase  SetLabelV=on  LabelV=V22  Vpu=off  VpuLL=off  CurrentMeasurement=yes  SetLabelI=on  LabelI=I2221  Ipu=off  Pbase=100e6  Vbase=500e3  OutputType=Magnitude-Angle  PhasorSimulation=on  PSBequivalent=0
  I2221A : PMIOPort  Port=1  Side=Left
  I2221B : PMIOPort  Port=2  Side=Left
  I2221C : PMIOPort  Port=3  Side=Left
  I2224A : PMIOPort  Port=4  Side=Right
  I2224B : PMIOPort  Port=5  Side=Right
  I2224C : PMIOPort  Port=6  Side=Right
  I2210A : PMIOPort  Port=7  Side=Left
  I2210B : PMIOPort  Port=8  Side=Left
  I2210C : PMIOPort  Port=9  Side=Left
  wires:
  [V22] -> To Workspace6/1
  [I2221] -> To Workspace2/1
  [I2210] -> To Workspace1/1
  [I2224] -> To Workspace3/1
  connections:
  V22 I2221/RConn2 -- I2221B/RConn1
  I2210/RConn1 -- I2210A/RConn1
  V22 I2221/RConn1 -- I2221A/RConn1
  I2210/RConn2 -- I2210B/RConn1
  I2210/RConn3 -- I2210C/RConn1
  V22 I2221/RConn3 -- I2221C/RConn1
  V22 I2221/LConn1 -- I2224/LConn1 -- I2210/LConn1
  V22 I2221/LConn2 -- I2224/LConn2 -- I2210/LConn2
  V22 I2221/LConn3 -- I2224/LConn3 -- I2210/LConn3
  I2224/RConn1 -- I2224A/RConn1
  I2224/RConn2 -- I2224B/RConn1
  I2224/RConn3 -- I2224C/RConn1

== system ieee30/Bus23 ==
  I2324 : powerlib/Measurements/Three-Phase V-I Measurement  VoltageMeasurement=no  SetLabelV=off  LabelV=Vabc  Vpu=off  VpuLL=off  CurrentMeasurement=yes  SetLabelI=on  LabelI=I2324  Ipu=off  Pbase=100e6  Vbase=500e3  OutputType=Magnitude-Angle  PhasorSimulation=on  PSBequivalent=0
  Load23 : powerlib/Measurements/Three-Phase V-I Measurement  VoltageMeasurement=no  SetLabelV=off  LabelV=V21  Vpu=off  VpuLL=off  CurrentMeasurement=no  SetLabelI=off  LabelI=I2224  Ipu=off  Pbase=100e6  Vbase=500e3  OutputType=Complex  PhasorSimulation=on  PSBequivalent=0
  To Workspace1 : ToWorkspace  VariableName=V23  SaveFormat=Timeseries  SampleTime=0.01
  To Workspace2 : ToWorkspace  VariableName=I2315  SaveFormat=Timeseries  SampleTime=0.01
  To Workspace3 : ToWorkspace  VariableName=I2324  SaveFormat=Timeseries  SampleTime=0.01
  V23 I2315 : powerlib/Measurements/Three-Phase V-I Measurement  VoltageMeasurement=phase-to-phase  SetLabelV=on  LabelV=V23  Vpu=off  VpuLL=off  CurrentMeasurement=yes  SetLabelI=on  LabelI=I2315  Ipu=off  Pbase=100e6  Vbase=500e3  OutputType=Magnitude-Angle  PhasorSimulation=on  PSBequivalent=0
  I2315A : PMIOPort  Port=1  Side=Left
  I2315B : PMIOPort  Port=2  Side=Left
  I2315C : PMIOPort  Port=3  Side=Left
  Load23A : PMIOPort  Port=4  Side=Right
  Load23B : PMIOPort  Port=5  Side=Right
  Load23C : PMIOPort  Port=6  Side=Right
  I2324A : PMIOPort  Port=7  Side=Left
  I2324B : PMIOPort  Port=8  Side=Left
  I2324C : PMIOPort  Port=9  Side=Left
  wires:
  [V23] -> To Workspace1/1
  [I2315] -> To Workspace2/1
  [I2324] -> To Workspace3/1
  connections:
  V23 I2315/RConn2 -- I2315B/RConn1
  I2324/RConn1 -- I2324A/RConn1
  V23 I2315/RConn1 -- I2315A/RConn1
  I2324/RConn2 -- I2324B/RConn1
  I2324/RConn3 -- I2324C/RConn1
  V23 I2315/RConn3 -- I2315C/RConn1
  V23 I2315/LConn1 -- Load23/LConn1 -- I2324/LConn1
  V23 I2315/LConn2 -- Load23/LConn2 -- I2324/LConn2
  V23 I2315/LConn3 -- Load23/LConn3 -- I2324/LConn3
  Load23/RConn1 -- Load23A/RConn1
  Load23/RConn2 -- Load23B/RConn1
  Load23/RConn3 -- Load23C/RConn1

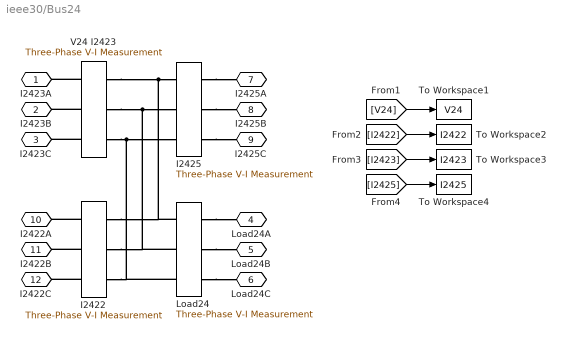
== system ieee30/Bus24 ==
  I2422 : powerlib/Measurements/Three-Phase V-I Measurement  VoltageMeasurement=no  SetLabelV=off  LabelV=V24  Vpu=off  VpuLL=off  CurrentMeasurement=yes  SetLabelI=on  LabelI=I2422  Ipu=off  Pbase=100e6  Vbase=500e3  OutputType=Magnitude-Angle  PhasorSimulation=on  PSBequivalent=0
  I2425 : powerlib/Measurements/Three-Phase V-I Measurement  VoltageMeasurement=no  SetLabelV=off  LabelV=Vabc  Vpu=off  VpuLL=off  CurrentMeasurement=yes  SetLabelI=on  LabelI=I2425  Ipu=off  Pbase=100e6  Vbase=500e3  OutputType=Magnitude-Angle  PhasorSimulation=on  PSBequivalent=0
  Load24 : powerlib/Measurements/Three-Phase V-I Measurement  VoltageMeasurement=no  SetLabelV=off  LabelV=V21  Vpu=off  VpuLL=off  CurrentMeasurement=no  SetLabelI=off  LabelI=I2224  Ipu=off  Pbase=100e6  Vbase=500e3  OutputType=Complex  PhasorSimulation=on  PSBequivalent=0
  To Workspace1 : ToWorkspace  VariableName=V24  SaveFormat=Timeseries  SampleTime=0.01
  To Workspace2 : ToWorkspace  VariableName=I2422  SaveFormat=Timeseries  SampleTime=0.01
  To Workspace3 : ToWorkspace  VariableName=I2423  SaveFormat=Timeseries  SampleTime=0.01
  To Workspace4 : ToWorkspace  VariableName=I2425  SaveFormat=Timeseries  SampleTime=0.01
  V24 I2423 : powerlib/Measurements/Three-Phase V-I Measurement  VoltageMeasurement=phase-to-phase  SetLabelV=on  LabelV=V24  Vpu=off  VpuLL=off  CurrentMeasurement=yes  SetLabelI=on  LabelI=I2423  Ipu=off  Pbase=100e6  Vbase=500e3  OutputType=Magnitude-Angle  PhasorSimulation=on  PSBequivalent=0
  I2423A : PMIOPort  Port=1  Side=Left
  I2423B : PMIOPort  Port=2  Side=Left
  I2423C : PMIOPort  Port=3  Side=Left
  Load24A : PMIOPort  Port=4  Side=Right
  Load24B : PMIOPort  Port=5  Side=Right
  Load24C : PMIOPort  Port=6  Side=Right
  I2425A : PMIOPort  Port=7  Side=Right
  I2425B : PMIOPort  Port=8  Side=Right
  I2425C : PMIOPort  Port=9  Side=Right
  I2422A : PMIOPort  Port=10  Side=Left
  I2422B : PMIOPort  Port=11  Side=Left
  I2422C : PMIOPort  Port=12  Side=Left
  wires:
  [V24] -> To Workspace1/1
  [I2422] -> To Workspace2/1
  [I2423] -> To Workspace3/1
  [I2425] -> To Workspace4/1
  connections:
  V24 I2423/RConn2 -- I2423B/RConn1
  I2425/RConn1 -- I2425A/RConn1
  V24 I2423/RConn1 -- I2423A/RConn1
  I2425/RConn2 -- I2425B/RConn1
  I2425/RConn3 -- I2425C/RConn1
  V24 I2423/RConn3 -- I2423C/RConn1
  V24 I2423/LConn1 -- I2422/LConn1 -- Load24/LConn1 -- I2425/LConn1
  V24 I2423/LConn2 -- Load24/LConn2 -- I2422/LConn2 -- I2425/LConn2
  V24 I2423/LConn3 -- Load24/LConn3 -- I2422/LConn3 -- I2425/LConn3
  Load24/RConn1 -- Load24A/RConn1
  Load24/RConn2 -- Load24B/RConn1
  Load24/RConn3 -- Load24C/RConn1
  I2422/RConn1 -- I2422A/RConn1
  I2422/RConn2 -- I2422B/RConn1
  I2422/RConn3 -- I2422C/RConn1

== system ieee30/Bus25 ==
  I2526 : powerlib/Measurements/Three-Phase V-I Measurement  VoltageMeasurement=no  SetLabelV=off  LabelV=Vabc  Vpu=off  VpuLL=off  CurrentMeasurement=yes  SetLabelI=on  LabelI=I2526  Ipu=off  Pbase=100e6  Vbase=500e3  OutputType=Magnitude-Angle  PhasorSimulation=on  PSBequivalent=0
  I2527 : powerlib/Measurements/Three-Phase V-I Measurement  VoltageMeasurement=no  SetLabelV=off  LabelV=V21  Vpu=off  VpuLL=off  CurrentMeasurement=yes  SetLabelI=on  LabelI=I2527  Ipu=off  Pbase=100e6  Vbase=500e3  OutputType=Magnitude-Angle  PhasorSimulation=on  PSBequivalent=0
  To Workspace1 : ToWorkspace  VariableName=V25  SaveFormat=Timeseries  SampleTime=0.01
  To Workspace2 : ToWorkspace  VariableName=I2524  SaveFormat=Timeseries  SampleTime=0.01
  To Workspace3 : ToWorkspace  VariableName=I2526  SaveFormat=Timeseries  SampleTime=0.01
  To Workspace4 : ToWorkspace  VariableName=I2527  SaveFormat=Timeseries  SampleTime=0.01
  V25 I2524 : powerlib/Measurements/Three-Phase V-I Measurement  VoltageMeasurement=phase-to-phase  SetLabelV=on  LabelV=V25  Vpu=off  VpuLL=off  CurrentMeasurement=yes  SetLabelI=on  LabelI=I2524  Ipu=off  Pbase=100e6  Vbase=500e3  OutputType=Magnitude-Angle  PhasorSimulation=on  PSBequivalent=0
  I2524A : PMIOPort  Port=1  Side=Left
  I2524B : PMIOPort  Port=2  Side=Left
  I2524C : PMIOPort  Port=3  Side=Left
  I2527A : PMIOPort  Port=4  Side=Right
  I2527B : PMIOPort  Port=5  Side=Right
  I2527C : PMIOPort  Port=6  Side=Right
  I2526A : PMIOPort  Port=7  Side=Left
  I2526B : PMIOPort  Port=8  Side=Left
  I2526C : PMIOPort  Port=9  Side=Left
  wires:
  [V25] -> To Workspace1/1
  [I2524] -> To Workspace2/1
  [I2526] -> To Workspace3/1
  [I2527] -> To Workspace4/1
  connections:
  V25 I2524/RConn2 -- I2524B/RConn1
  I2526/RConn1 -- I2526A/RConn1
  V25 I2524/RConn1 -- I2524A/RConn1
  I2526/RConn2 -- I2526B/RConn1
  I2526/RConn3 -- I2526C/RConn1
  V25 I2524/RConn3 -- I2524C/RConn1
  V25 I2524/LConn1 -- I2527/LConn1 -- I2526/LConn1
  V25 I2524/LConn2 -- I2527/LConn2 -- I2526/LConn2
  V25 I2524/LConn3 -- I2527/LConn3 -- I2526/LConn3
  I2527/RConn1 -- I2527A/RConn1
  I2527/RConn2 -- I2527B/RConn1
  I2527/RConn3 -- I2527C/RConn1

== system ieee30/Bus26 ==
  Load26 : powerlib/Measurements/Three-Phase V-I Measurement  VoltageMeasurement=no  SetLabelV=off  LabelV=Vabc  Vpu=off  VpuLL=off  CurrentMeasurement=no  SetLabelI=off  LabelI=Iabc  Ipu=off  Pbase=100e6  Vbase=500e3  OutputType=Complex  PhasorSimulation=on  PSBequivalent=0
  To Workspace1 : ToWorkspace  VariableName=V26  SaveFormat=Timeseries  SampleTime=0.01
  To Workspace2 : ToWorkspace  VariableName=I2625  SaveFormat=Timeseries  SampleTime=0.01
  V26 I2625 : powerlib/Measurements/Three-Phase V-I Measurement  VoltageMeasurement=phase-to-phase  SetLabelV=on  LabelV=V26  Vpu=off  VpuLL=off  CurrentMeasurement=yes  SetLabelI=on  LabelI=I2625  Ipu=off  Pbase=100e6  Vbase=500e3  OutputType=Magnitude-Angle  PhasorSimulation=on  PSBequivalent=0
  I2625A : PMIOPort  Port=1  Side=Left
  I2625B : PMIOPort  Port=2  Side=Left
  I2625C : PMIOPort  Port=3  Side=Left
  Load26A : PMIOPort  Port=4  Side=Right
  Load26B : PMIOPort  Port=5  Side=Right
  Load26C : PMIOPort  Port=6  Side=Right
  wires:
  [V26] -> To Workspace1/1
  [I2625] -> To Workspace2/1
  connections:
  V26 I2625/RConn3 -- I2625C/RConn1
  V26 I2625/RConn2 -- I2625B/RConn1
  V26 I2625/RConn1 -- I2625A/RConn1
  Load26/RConn2 -- Load26B/RConn1
  Load26/RConn1 -- Load26A/RConn1
  Load26/RConn3 -- Load26C/RConn1
  Load26/LConn1 -- V26 I2625/LConn1
  Load26/LConn2 -- V26 I2625/LConn2
  Load26/LConn3 -- V26 I2625/LConn3

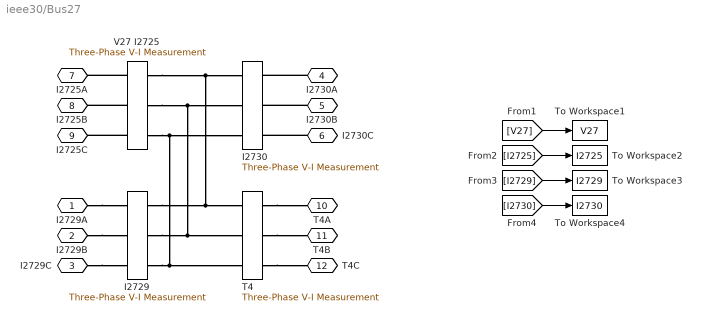
== system ieee30/Bus27 ==
  I2729 : powerlib/Measurements/Three-Phase V-I Measurement  VoltageMeasurement=no  SetLabelV=off  LabelV=V27  Vpu=off  VpuLL=off  CurrentMeasurement=yes  SetLabelI=on  LabelI=I2729  Ipu=off  Pbase=100e6  Vbase=500e3  OutputType=Magnitude-Angle  PhasorSimulation=on  PSBequivalent=0
  I2730 : powerlib/Measurements/Three-Phase V-I Measurement  VoltageMeasurement=no  SetLabelV=off  LabelV=V27  Vpu=off  VpuLL=off  CurrentMeasurement=yes  SetLabelI=on  LabelI=I2730  Ipu=off  Pbase=100e6  Vbase=500e3  OutputType=Magnitude-Angle  PhasorSimulation=on  PSBequivalent=0
  T4 : powerlib/Measurements/Three-Phase V-I Measurement  VoltageMeasurement=no  SetLabelV=off  LabelV=V27  Vpu=off  VpuLL=off  CurrentMeasurement=no  SetLabelI=off  LabelI=I2730  Ipu=off  Pbase=100e6  Vbase=500e3  OutputType=Complex  PhasorSimulation=on  PSBequivalent=0
  To Workspace1 : ToWorkspace  VariableName=V27  SaveFormat=Timeseries  SampleTime=0.01
  To Workspace2 : ToWorkspace  VariableName=I2725  SaveFormat=Timeseries  SampleTime=0.01
  To Workspace3 : ToWorkspace  VariableName=I2729  SaveFormat=Timeseries  SampleTime=0.01
  To Workspace4 : ToWorkspace  VariableName=I2730  SaveFormat=Timeseries  SampleTime=0.01
  V27 I2725 : powerlib/Measurements/Three-Phase V-I Measurement  VoltageMeasurement=phase-to-phase  SetLabelV=on  LabelV=V27  Vpu=off  VpuLL=off  CurrentMeasurement=yes  SetLabelI=on  LabelI=I2725  Ipu=off  Pbase=100e6  Vbase=500e3  OutputType=Magnitude-Angle  PhasorSimulation=on  PSBequivalent=0
  I2729A : PMIOPort  Port=1  Side=Left
  I2729B : PMIOPort  Port=2  Side=Left
  I2729C : PMIOPort  Port=3  Side=Left
  I2730A : PMIOPort  Port=4  Side=Left
  I2730B : PMIOPort  Port=5  Side=Left
  I2730C : PMIOPort  Port=6  Side=Left
  I2725A : PMIOPort  Port=7  Side=Left
  I2725B : PMIOPort  Port=8  Side=Left
  I2725C : PMIOPort  Port=9  Side=Left
  T4A : PMIOPort  Port=10  Side=Right
  T4B : PMIOPort  Port=11  Side=Right
  T4C : PMIOPort  Port=12  Side=Right
  wires:
  [V27] -> To Workspace1/1
  [I2725] -> To Workspace2/1
  [I2729] -> To Workspace3/1
  [I2730] -> To Workspace4/1
  connections:
  V27 I2725/RConn3 -- I2725C/RConn1
  T4/RConn1 -- T4A/RConn1
  T4/RConn3 -- T4C/RConn1
  T4/RConn2 -- T4B/RConn1
  V27 I2725/RConn2 -- I2725B/RConn1
  V27 I2725/RConn1 -- I2725A/RConn1
  V27 I2725/LConn1 -- I2730/LConn1 -- T4/LConn1 -- I2729/LConn1
  V27 I2725/LConn2 -- T4/LConn2 -- I2729/LConn2 -- I2730/LConn2
  V27 I2725/LConn3 -- T4/LConn3 -- I2729/LConn3 -- I2730/LConn3
  I2729B/RConn1 -- I2729/RConn2
  I2729A/RConn1 -- I2729/RConn1
  I2729C/RConn1 -- I2729/RConn3
  I2730A/RConn1 -- I2730/RConn1
  I2730B/RConn1 -- I2730/RConn2
  I2730C/RConn1 -- I2730/RConn3

== system ieee30/Bus28 ==
  I288 : powerlib/Measurements/Three-Phase V-I Measurement  VoltageMeasurement=no  SetLabelV=off  LabelV=Vabc  Vpu=off  VpuLL=off  CurrentMeasurement=yes  SetLabelI=on  LabelI=I288  Ipu=off  Pbase=100e6  Vbase=500e3  OutputType=Magnitude-Angle  PhasorSimulation=on  PSBequivalent=0
  T4 : powerlib/Measurements/Three-Phase V-I Measurement  VoltageMeasurement=no  SetLabelV=off  LabelV=V21  Vpu=off  VpuLL=off  CurrentMeasurement=no  SetLabelI=off  LabelI=I2224  Ipu=off  Pbase=100e6  Vbase=500e3  OutputType=Complex  PhasorSimulation=on  PSBequivalent=0
  To Workspace1 : ToWorkspace  VariableName=V28  SaveFormat=Timeseries  SampleTime=0.01
  To Workspace2 : ToWorkspace  VariableName=I286  SaveFormat=Timeseries  SampleTime=0.01
  To Workspace3 : ToWorkspace  VariableName=I288  SaveFormat=Timeseries  SampleTime=0.01
  V28 I286 : powerlib/Measurements/Three-Phase V-I Measurement  VoltageMeasurement=phase-to-phase  SetLabelV=on  LabelV=V28  Vpu=off  VpuLL=off  CurrentMeasurement=yes  SetLabelI=on  LabelI=I286  Ipu=off  Pbase=100e6  Vbase=500e3  OutputType=Magnitude-Angle  PhasorSimulation=on  PSBequivalent=0
  I288C : PMIOPort  Port=1  Side=Right
  I288B : PMIOPort  Port=2  Side=Right
  I288A : PMIOPort  Port=3  Side=Right
  I286C : PMIOPort  Port=4  Side=Right
  I286B : PMIOPort  Port=5  Side=Right
  I286A : PMIOPort  Port=6  Side=Right
  T4A : PMIOPort  Port=7  Side=Left
  T4B : PMIOPort  Port=8  Side=Left
  T4C : PMIOPort  Port=9  Side=Left
  wires:
  [V28] -> To Workspace1/1
  [I286] -> To Workspace2/1
  [I288] -> To Workspace3/1
  connections:
  V28 I286/RConn2 -- I286B/RConn1
  I288/RConn1 -- I288A/RConn1
  V28 I286/RConn1 -- I286A/RConn1
  I288/RConn2 -- I288B/RConn1
  I288/RConn3 -- I288C/RConn1
  V28 I286/RConn3 -- I286C/RConn1
  V28 I286/LConn1 -- T4/LConn1 -- I288/LConn1
  V28 I286/LConn2 -- T4/LConn2 -- I288/LConn2
  V28 I286/LConn3 -- T4/LConn3 -- I288/LConn3
  T4/RConn1 -- T4A/RConn1
  T4/RConn2 -- T4B/RConn1
  T4/RConn3 -- T4C/RConn1
